simulink model "process"  (R2018b)
settings: Solver=VariableStepAuto  StartTime=0.0  StopTime=10.0  RelTol=1e-3
settings Model: Creator=jh2044  LastModifiedBy=jh2044

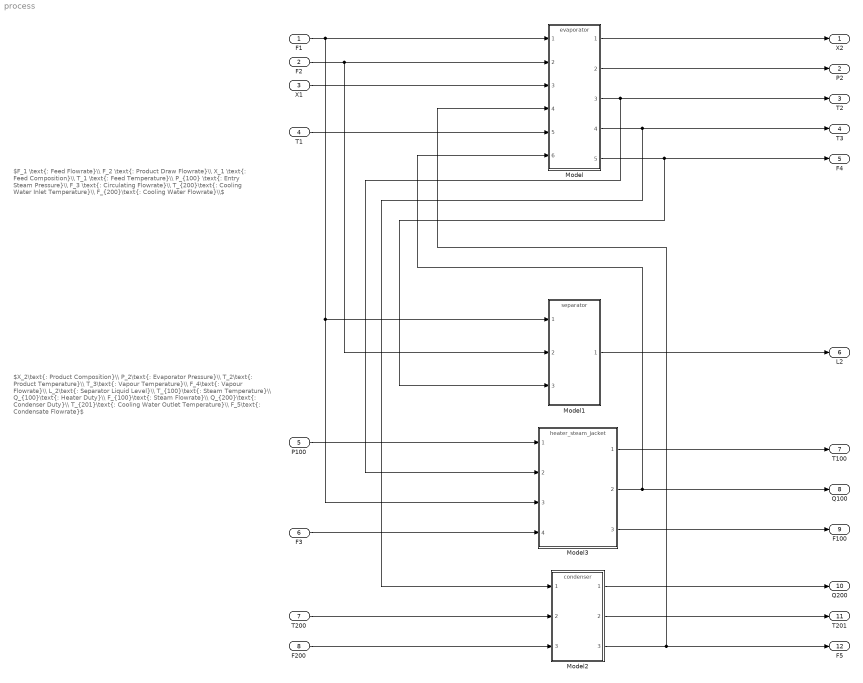
== system process ==
  note: $X_2\text{: Product Composition}\\ P_2\text{: Evaporator Pressure}\\ T_2\text{: Product Temperature}\\ T_3\text{: Vapour Temperature}\\ F_4\text{: Vapour Flowrate}\\ L_2\text{: Separator Liquid Level}\\ T_{100}\text{: Steam Temperature}\\ Q_{100}\text{: Heater Duty}\\ F_{100}\text{: Steam Flowrate}\\ Q_{200}\text{: Condenser Duty}\\ T_{201}\text{: Cooling Water Outlet Temperature}\\ F_5\text{: Condensate Flowrate}$
  note: $F_1 \text{: Feed Flowrate}\\ F_2 \text{: Product Draw Flowrate}\\ X_1 \text{: Feed Composition}\\ T_1 \text{: Feed Temperature}\\ P_{100} \text{: Entry Steam Pressure}\\ F_3 \text{: Circulating Flowrate}\\ T_{200}\text{: Cooling Water Inlet Temperature}\\ F_{200}\text{: Cooling Water Flowrate}\\$
  F1 : Inport
  F2 : Inport  Port=2
  X1 : Inport  Port=3
  T1 : Inport  Port=4
  P100 : Inport  Port=5
  F3 : Inport  Port=6
  T200 : Inport  Port=7
  F200 : Inport  Port=8
  Model : ModelReference  ModelNameDialog=evaporator  SimulationMode=Normal  ModelReferenceVersion=1.4
  Model1 : ModelReference  ModelNameDialog=separator  SimulationMode=Normal  ModelReferenceVersion=1.1
  Model2 : ModelReference  ModelNameDialog=condenser  SimulationMode=Normal  ModelReferenceVersion=1.8
  Model3 : ModelReference  ModelNameDialog=heater_steam_jacket.slx  SimulationMode=Normal  ModelReferenceVersion=1.3
  X2 : Outport
  P2 : Outport  Port=2
  T2 : Outport  Port=3
  T3 : Outport  Port=4
  F4 : Outport  Port=5
  L2 : Outport  Port=6
  T100 : Outport  Port=7
  Q100 : Outport  Port=8
  F100 : Outport  Port=9
  Q200 : Outport  Port=10
  T201 : Outport  Port=11
  F5 : Outport  Port=12
  wires:
  F1/1 -> Model3/3, Model1/1, Model/1
  F2/1 -> Model1/2, Model/2
  X1/1 -> Model/3
  T1/1 -> Model/5
  Model/5 -> F4/1, Model1/3
  P100/1 -> Model3/1
  F3/1 -> Model3/4
  Model/1 -> X2/1
  Model/2 -> P2/1
  Model/3 -> T2/1, Model3/2
  Model/4 -> T3/1, Model2/1
  Model1/1 -> L2/1
  Model3/1 -> T100/1
  Model3/2 -> Model/6, Q100/1
  Model3/3 -> F100/1
  T200/1 -> Model2/2
  F200/1 -> Model2/3
  Model2/3 -> F5/1, Model/4
  Model2/1 -> Q200/1
  Model2/2 -> T201/1
